simulink model "EXP_Controller_SURGE"  (R2015b)
settings: Solver=VariableStepAuto  StartTime=0.0  StopTime=1000  RelTol=1e-3
values from neighbouring files (symbols this model uses):
  breakpoints1 = data(end:-1:1,1)'    [Experimental_Impl.m]    (also in Experimental_Impl_wPlot.m; FEB02_LAKE_TEST.m; FEB14_LAKE_TEST.m; FEB28_LAKE_TEST.m)
  drag_coeff = 16.91    [Experimental_Impl.m]    (also in Experimental_Impl_wPlot.m; FEB02_LAKE_TEST.m; FEB02_Post_Processing.m; FEB14_LAKE_TEST.m)
  Kds = .01    (= 0.01)    [Experimental_Impl.m]    (also in FEB02_LAKE_TEST.m = 1; FEB02_Post_Processing.m = Gain_S(3,i); FEB14_LAKE_TEST.m; FEB28_LAKE_TEST.m = 0)
  Kis = .1    (= 0.1)    [Experimental_Impl.m]    (also in FEB02_LAKE_TEST.m = 1; FEB02_Post_Processing.m = Gain_S(2,i); FEB14_LAKE_TEST.m = 7; FEB28_LAKE_TEST.m = 15)
  Kps = 1    [Experimental_Impl.m]    (also in FEB02_LAKE_TEST.m; FEB02_Post_Processing.m = Gain_S(1,i); FEB14_LAKE_TEST.m = 12; FEB28_LAKE_TEST.m = 40)
  switch_case = 0    [Experimental_Impl.m]    (also in Experimental_Impl_wPlot.m; FEB02_LAKE_TEST.m; FEB02_Post_Processing.m; FEB14_LAKE_TEST.m)
  table_data = data(end:-1:1,2)'    [Experimental_Impl.m]    (also in Experimental_Impl_wPlot.m; FEB02_LAKE_TEST.m; FEB14_LAKE_TEST.m; FEB28_LAKE_TEST.m)
  vf = 0.25    [Experimental_Impl.m]    (also in Experimental_Impl_wPlot.m = 0; FEB02_LAKE_TEST.m = 0; FEB02_Post_Processing.m = 1.25; FEB14_LAKE_TEST.m = 1.5)
  vo = 0.0    (= 0)    [Experimental_Impl.m]    (also in Experimental_Impl_wPlot.m; FEB02_LAKE_TEST.m; FEB02_Post_Processing.m = 1.25; FEB14_LAKE_TEST.m = 1.25)
  yf = pi()/4    [Experimental_Impl.m]    (also in Experimental_Impl_wPlot.m = 0; FEB02_LAKE_TEST.m = 0; FEB02_Post_Processing.m; FEB14_LAKE_TEST.m = 0)
  yo = 0    [Experimental_Impl.m]    (also in Experimental_Impl_wPlot.m; FEB02_LAKE_TEST.m; FEB02_Post_Processing.m; FEB14_LAKE_TEST.m)
undefined symbols (not defined in the file or in its folder): Left, Right
libraries: robotlib x3, realtime_pacer_lib x1
settings Model: Creator=bsb  LastModifiedBy=aschnieders22
settings ConfigComp: CovModelRefEnable=Off

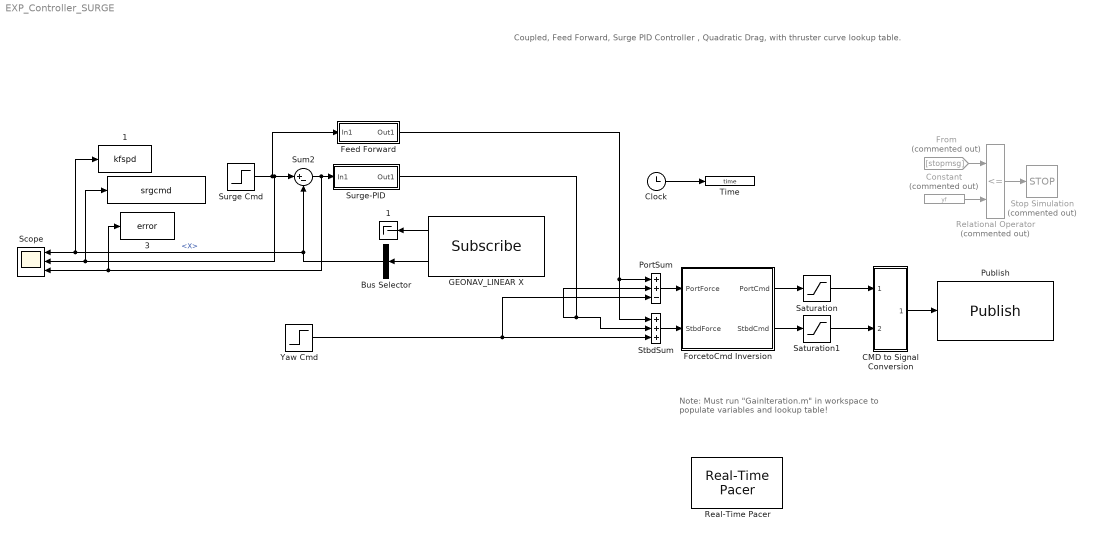
== system EXP_Controller_SURGE ==
  note: Note: Must run "GainIteration.m" in workspace to populate variables and lookup table!
  note: Coupled, Feed Forward, Surge PID Controller , Quadratic Drag, with thruster curve lookup table.
  " " : ToWorkspace  VariableName=srgcmd  SampleTime=-1
  " 1" : ToWorkspace  VariableName=kfspd  SampleTime=-1
  " 1" : Terminator
  " 3" : ToWorkspace  VariableName=error  SampleTime=-1
  Bus Selector : BusSelector  OutputSignals=Twist.Twist.Linear.X
  CMD to Signal Conversion : Subsystem
  Clock : Clock
  Constant : Constant  Commented=on  Value=yf
  Feed Forward : Subsystem
  ForcetoCmd Inversion : Subsystem
  From : From  Commented=on  GotoTag=stopmsg
  GEONAV_LINEAR X : robotlib/Subscribe  SourceLibraryInfo=This block requires Robotics System Toolbox  topicSource=Select from ROS network  topic=/geonav_odom  messageType=nav_msgs/Odometry  sampleTime=-1  messageQueueLength=1
  PortSum : Sum  Inputs=++-
  Publish : robotlib/Publish  SourceLibraryInfo=This block requires Robotics System Toolbox  topicSource=Select from ROS network  topic=/cmd_drive  messageType=kingfisher_msgs/Drive  messageQueueLength=1
  Real-Time Pacer : realtime_pacer_lib/Real-Time Pacer  simTimePerRealTime=1
  Relational Operator : RelationalOperator  Commented=on  Operator=<=  OutDataTypeStr=boolean
  Saturation : Saturate  UpperLimit=1  LowerLimit=-1
  Saturation1 : Saturate  UpperLimit=1  LowerLimit=-1
  Scope : Scope  NumInputPorts=3
  StbdSum : Sum  Inputs=+++
  Stop Simulation : Stop  Commented=on
  Sum2 : Sum  Inputs=|+-
  Surge Cmd : Step  Time=10  Before=vo  After=vf  SampleTime=0
  Surge-PID : Subsystem
  Time : ToWorkspace  VariableName=time  SampleTime=-1
  Yaw Cmd : Step  Time=20  Before=yo  After=yf  SampleTime=0
  wires:
  Clock/1 -> Time/1
  PortSum/1 -> ForcetoCmd Inversion/1(PortForce)
  StbdSum/1 -> ForcetoCmd Inversion/2(StbdForce)
  Surge Cmd/1 -> " "/1, Scope/2, Sum2/1, Feed Forward/1(In1)
  Sum2/1 -> " 3"/1, Scope/3, Surge-PID/1(In1)
  Surge-PID/1(Out1) -> PortSum/2, StbdSum/2
  Relational Operator/1 -> Stop Simulation/1
  Constant/1 -> Relational Operator/2
  From/1 -> Relational Operator/1
  Saturation1/1 -> CMD to Signal Conversion/2(In2)
  Saturation/1 -> CMD to Signal Conversion/1(In1)
  ForcetoCmd Inversion/1(PortCmd) -> Saturation/1
  ForcetoCmd Inversion/2(StbdCmd) -> Saturation1/1
  CMD to Signal Conversion/1(Out1) -> Publish/1
  Feed Forward/1(Out1) -> PortSum/1, StbdSum/1
  GEONAV_LINEAR X/1 -> " 1"/1
  GEONAV_LINEAR X/2 -> Bus Selector/1
  Bus Selector/1 -> Sum2/2, " 1"/1, Scope/1  "<X>"
  Yaw Cmd/1 -> PortSum/3, StbdSum/3

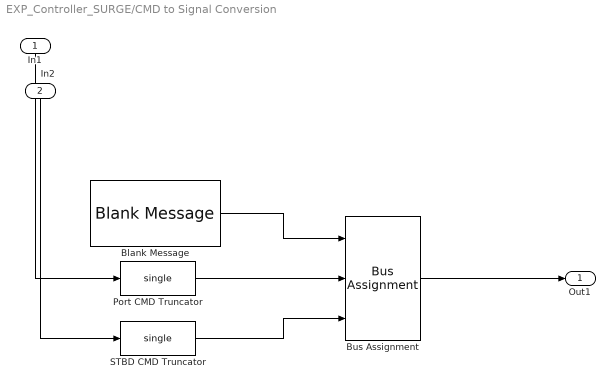
== system EXP_Controller_SURGE/CMD to Signal Conversion ==
  In1 : Inport
  In2 : Inport  Port=2
  Blank Message : robotlib/Blank Message  SourceLibraryInfo=This block requires Robotics System Toolbox  messageType=kingfisher_msgs/Drive  SampleTime=inf
  Bus Assignment : BusAssignment  AssignedSignals=Left,Right
  Port CMD Truncator : DataTypeConversion  OutDataTypeStr=single
  STBD CMD Truncator : DataTypeConversion  OutDataTypeStr=single
  Out1 : Outport
  wires:
  In2/1 -> STBD CMD Truncator/1
  In1/1 -> Port CMD Truncator/1
  Bus Assignment/1 -> Out1/1
  Blank Message/1 -> Bus Assignment/1
  Port CMD Truncator/1 -> Bus Assignment/2
  STBD CMD Truncator/1 -> Bus Assignment/3

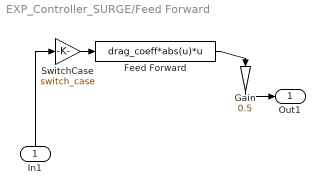
== system EXP_Controller_SURGE/Feed Forward ==
  In1 : Inport
  Feed Forward : Fcn  Expr=drag_coeff*abs(u)*u
  Gain : Gain  Gain=0.5
  SwitchCase : Gain  Gain=switch_case
  Out1 : Outport
  wires:
  In1/1 -> SwitchCase/1
  SwitchCase/1 -> Feed Forward/1
  Feed Forward/1 -> Gain/1
  Gain/1 -> Out1/1

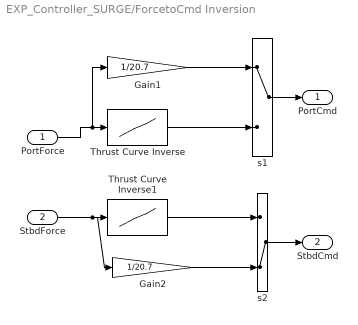
== system EXP_Controller_SURGE/ForcetoCmd Inversion ==
  PortForce : Inport
  StbdForce : Inport  Port=2
  Gain1 : Gain  Gain=1/20.7
  Gain2 : Gain  Gain=1/20.7
  Thrust Curve Inverse : Lookup_n-D  NumberOfTableDimensions=1  BreakpointsForDimension1=table_data  Table=breakpoints1  ExtrapMethod=Clip  UseLastTableValue=on  InternalRulePriority=Speed  RndMeth=Simplest  InputSameDT=on
  Thrust Curve Inverse1 : Lookup_n-D  NumberOfTableDimensions=1  BreakpointsForDimension1=table_data  Table=breakpoints1  ExtrapMethod=Clip  UseLastTableValue=on  InternalRulePriority=Speed  RndMeth=Simplest  InputSameDT=on
  "s1 " : ManualSwitch
  s2 : ManualSwitch  CurrentSetting=0
  PortCmd : Outport
  StbdCmd : Outport  Port=2
  wires:
  StbdForce/1 -> Gain2/1, Thrust Curve Inverse1/1
  PortForce/1 -> Gain1/1, Thrust Curve Inverse/1
  Thrust Curve Inverse/1 -> "s1 "/2
  Gain1/1 -> "s1 "/1
  "s1 "/1 -> PortCmd/1
  s2/1 -> StbdCmd/1
  Thrust Curve Inverse1/1 -> s2/1
  Gain2/1 -> s2/2

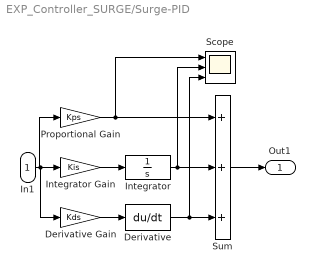
== system EXP_Controller_SURGE/Surge-PID ==
  In1 : Inport
  Derivative : Derivative  CoefficientInTFapproximation=0
  Derivative Gain : Gain  Gain=Kds
  Integrator : TransferFcn  Denominator=[1 0]
  Integrator Gain : Gain  Gain=Kis
  Proportional Gain : Gain  Gain=Kps
  Scope : Scope  NumInputPorts=3
  Sum : Sum  Inputs=+++
  Out1 : Outport
  wires:
  Derivative Gain/1 -> Derivative/1
  Integrator Gain/1 -> Integrator/1
  Derivative/1 -> Scope/3, Sum/3
  Sum/1 -> Out1/1
  Integrator/1 -> Scope/2, Sum/2
  Proportional Gain/1 -> Scope/1, Sum/1
  In1/1 -> Derivative Gain/1, Integrator Gain/1, Proportional Gain/1
